simulink model "plantaDrone5"  (R2021b)
settings: Solver=VariableStepAuto  StartTime=0.0  StopTime=2  RelTol=1e-3
values from neighbouring files (symbols this model uses):
  int5 = [0.0001,0.0001,0.0001,0.0001,0.0001,0.0001,0.0001,0.0001,0.0001,0.0001]    [linealControl.m]    (also in linealYcontrol5.m)
undefined symbols (not defined in the file or in its folder): lineal5simu
settings Model: Creator=LENOVO  LastModifiedBy=LENOVO

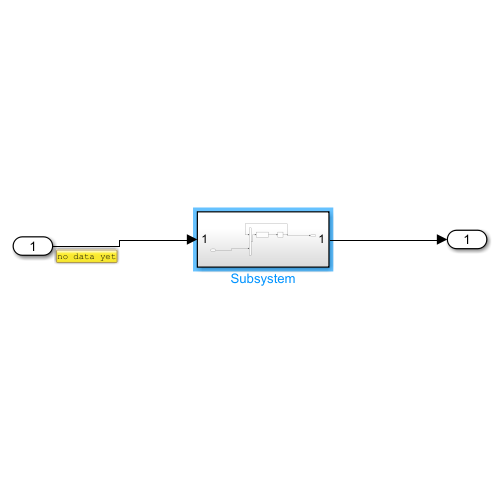
[thumbnail: Simulink's stored preview of the top-level diagram]
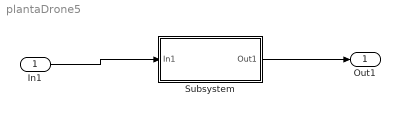
== system plantaDrone5 ==
  In1 : Inport
  Subsystem : Subsystem
  Out1 : Outport
  wires:
  In1/1 -> Subsystem/1(In1)
  Subsystem/1(Out1) -> Out1/1

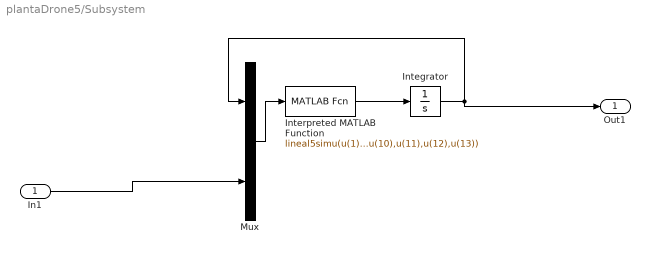
== system plantaDrone5/Subsystem ==
  In1 : Inport
  Integrator : Integrator  InitialCondition=int5
  Interpreted MATLAB Function : MATLABFcn  MATLABFcn=lineal5simu(u(1),u(2),u(3),u(4),u(5),u(6),u(7),u(8),u(9),u(10),u(11),u(12),u(13))
  Mux : Mux  Inputs=[10 3]
  Out1 : Outport
  wires:
  Interpreted MATLAB Function/1 -> Integrator/1
  Integrator/1 -> Mux/1, Out1/1
  Mux/1 -> Interpreted MATLAB Function/1
  In1/1 -> Mux/2
